simulink subsystem "rss_PwrTubPCBTempSensFaltDia"  (R2023a)
settings: Solver=VariableStepAuto  StartTime=0.0  StopTime=10.0  RelTol=1e-3
undefined symbols (not defined in the file): ENM_TYPE_FALT, Gu16_ctPCBTempFaltConfCnt_C, Gu16_ctPCBTempFaltRcvyCnt_C, Gu16_ctPwrTubTempFaltConfCnt_C, Gu16_ctPwrTubTempFaltRcvyCnt_C, Gu16_uADPCBTempFaltLoLim_C, Gu16_uADPwrTubTempFaltLoLim_C, Gu8_tNTCTempSensNoOpnCir_C, Gu8_tNTCTempSensOpnCir_C
libraries: lib_debounce x2, lib_configurable_parameter x2, lib_fault_definiteness x1
settings Model: Creator=xiaoqiang.yuan  LastModifiedBy=xiaoqiang.yuan

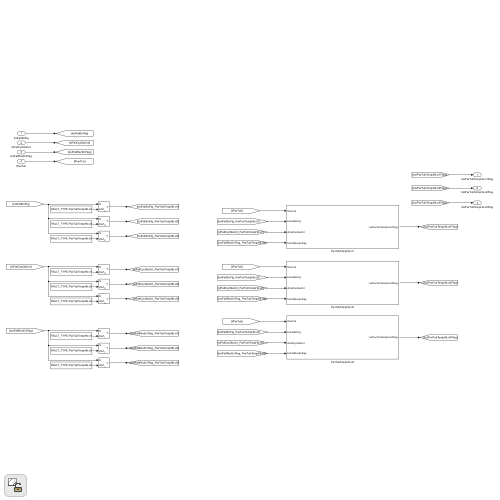
[thumbnail: Simulink's stored preview of the top-level diagram]
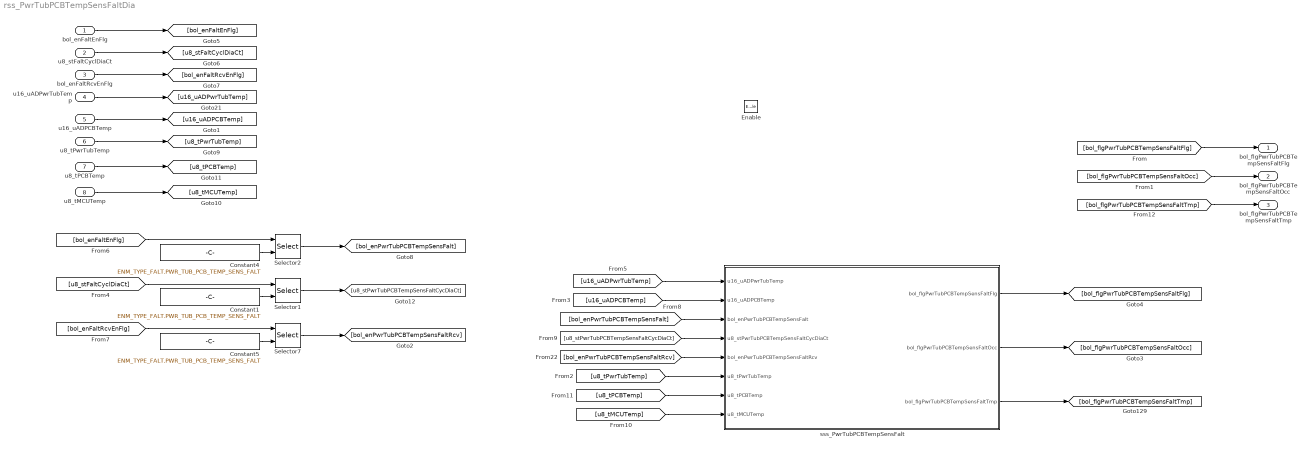
== system rss_PwrTubPCBTempSensFaltDia ==
  bol_enFaltEnFlg : Inport  OutDataTypeStr=boolean
  u8_stFaltCyclDiaCt : Inport  Port=2  OutDataTypeStr=uint8
  bol_enFaltRcvEnFlg : Inport  Port=3  OutDataTypeStr=boolean
  u16_uADPwrTubTemp : Inport  Port=4  OutDataTypeStr=uint16
  u16_uADPCBTemp : Inport  Port=5  OutDataTypeStr=uint16
  u8_tPwrTubTemp : Inport  Port=6  OutDataTypeStr=dt_Temp_u8p0bn40
  u8_tPCBTemp : Inport  Port=7  OutDataTypeStr=dt_Temp_u8p0bn40
  u8_tMCUTemp : Inport  Port=8  OutDataTypeStr=dt_Temp_u8p0bn40
  Enable : EnablePort
  Constant1 : Constant  Value=ENM_TYPE_FALT.PWR_TUB_PCB_TEMP_SENS_FALT
  Constant4 : Constant  Value=ENM_TYPE_FALT.PWR_TUB_PCB_TEMP_SENS_FALT
  Constant5 : Constant  Value=ENM_TYPE_FALT.PWR_TUB_PCB_TEMP_SENS_FALT
  Selector1 : Selector  IndexMode=Zero-based  InputPortWidth=Cdbl_numFaltDiaNum  IndexOptions=Index vector (port)  Indices=[1 3]  OutputSizes=1
  Selector2 : Selector  IndexMode=Zero-based  InputPortWidth=Cdbl_numFaltDiaNum  IndexOptions=Index vector (port)  Indices=[1 3]  OutputSizes=1
  Selector7 : Selector  IndexMode=Zero-based  InputPortWidth=Cdbl_numFaltDiaNum  IndexOptions=Index vector (port)  Indices=[1 3]  OutputSizes=1
  sss_PwrTubPCBTempSensFalt : Subsystem
  bol_flgPwrTubPCBTempSensFaltFlg : Outport  OutDataTypeStr=boolean
  bol_flgPwrTubPCBTempSensFaltOcc : Outport  Port=2  OutDataTypeStr=boolean
  bol_flgPwrTubPCBTempSensFaltTmp : Outport  Port=3  OutDataTypeStr=boolean
  wires:
  [bol_flgPwrTubPCBTempSensFaltFlg] -> bol_flgPwrTubPCBTempSensFaltFlg/1
  u16_uADPwrTubTemp/1 -> [u16_uADPwrTubTemp]
  Selector2/1 -> [bol_enPwrTubPCBTempSensFalt]
  [bol_enFaltEnFlg] -> Selector2/1
  [bol_enPwrTubPCBTempSensFalt] -> sss_PwrTubPCBTempSensFalt/3(bol_enPwrTubPCBTempSensFalt)
  Constant4/1 -> Selector2/2
  [u8_stPwrTubPCBTempSensFaltCycDiaCt] -> sss_PwrTubPCBTempSensFalt/4(u8_stPwrTubPCBTempSensFaltCycDiaCt)
  [u16_uADPwrTubTemp] -> sss_PwrTubPCBTempSensFalt/1(u16_uADPwrTubTemp)
  bol_enFaltEnFlg/1 -> [bol_enFaltEnFlg]
  bol_enFaltRcvEnFlg/1 -> [bol_enFaltRcvEnFlg]
  u8_stFaltCyclDiaCt/1 -> [u8_stFaltCyclDiaCt]
  [bol_enPwrTubPCBTempSensFaltRcv] -> sss_PwrTubPCBTempSensFalt/5(bol_enPwrTubPCBTempSensFaltRcv)
  Selector1/1 -> [u8_stPwrTubPCBTempSensFaltCycDiaCt]
  Constant1/1 -> Selector1/2
  [u8_stFaltCyclDiaCt] -> Selector1/1
  Selector7/1 -> [bol_enPwrTubPCBTempSensFaltRcv]
  Constant5/1 -> Selector7/2
  [bol_enFaltRcvEnFlg] -> Selector7/1
  sss_PwrTubPCBTempSensFalt/1(bol_flgPwrTubPCBTempSensFaltFlg) -> [bol_flgPwrTubPCBTempSensFaltFlg]
  u16_uADPCBTemp/1 -> [u16_uADPCBTemp]
  [u16_uADPCBTemp] -> sss_PwrTubPCBTempSensFalt/2(u16_uADPCBTemp)
  sss_PwrTubPCBTempSensFalt/2(bol_flgPwrTubPCBTempSensFaltOcc) -> [bol_flgPwrTubPCBTempSensFaltOcc]
  [bol_flgPwrTubPCBTempSensFaltOcc] -> bol_flgPwrTubPCBTempSensFaltOcc/1
  u8_tPCBTemp/1 -> [u8_tPCBTemp]
  u8_tMCUTemp/1 -> [u8_tMCUTemp]
  u8_tPwrTubTemp/1 -> [u8_tPwrTubTemp]
  [u8_tPwrTubTemp] -> sss_PwrTubPCBTempSensFalt/6(u8_tPwrTubTemp)
  [u8_tPCBTemp] -> sss_PwrTubPCBTempSensFalt/7(u8_tPCBTemp)
  [u8_tMCUTemp] -> sss_PwrTubPCBTempSensFalt/8(u8_tMCUTemp)
  [bol_flgPwrTubPCBTempSensFaltTmp] -> bol_flgPwrTubPCBTempSensFaltTmp/1
  sss_PwrTubPCBTempSensFalt/3(bol_flgPwrTubPCBTempSensFaltTmp) -> [bol_flgPwrTubPCBTempSensFaltTmp]

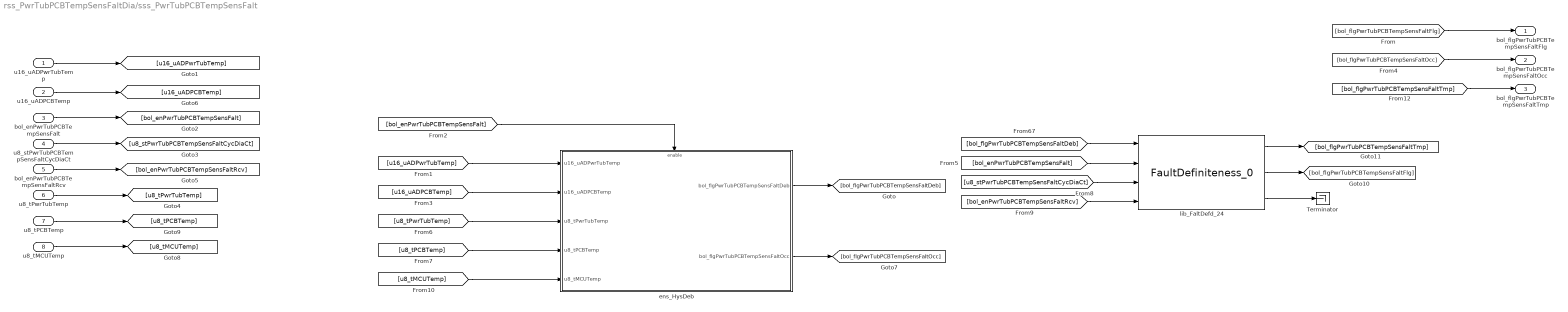
== system rss_PwrTubPCBTempSensFaltDia/sss_PwrTubPCBTempSensFalt ==
  u16_uADPwrTubTemp : Inport
  u16_uADPCBTemp : Inport  Port=2
  bol_enPwrTubPCBTempSensFalt : Inport  Port=3
  u8_stPwrTubPCBTempSensFaltCycDiaCt : Inport  Port=4
  bol_enPwrTubPCBTempSensFaltRcv : Inport  Port=5
  u8_tPwrTubTemp : Inport  Port=6
  u8_tPCBTemp : Inport  Port=7
  u8_tMCUTemp : Inport  Port=8
  Terminator : Terminator
  ens_HysDeb : Subsystem
  lib_FaltDefd_24 : lib_fault_definiteness/FaultDefiniteness_0  lb_FaltWaitRecvCnt=Gu16_ctPCBTempFaltConfCnt_C
  bol_flgPwrTubPCBTempSensFaltFlg : Outport
  bol_flgPwrTubPCBTempSensFaltOcc : Outport  Port=2
  bol_flgPwrTubPCBTempSensFaltTmp : Outport  Port=3  OutDataTypeStr=boolean
  wires:
  [bol_flgPwrTubPCBTempSensFaltTmp] -> bol_flgPwrTubPCBTempSensFaltTmp/1
  [u8_tMCUTemp] -> ens_HysDeb/5(u8_tMCUTemp)
  [u8_tPCBTemp] -> ens_HysDeb/4(u8_tPCBTemp)
  [u8_tPwrTubTemp] -> ens_HysDeb/3(u8_tPwrTubTemp)
  u8_tPCBTemp/1 -> [u8_tPCBTemp]
  u8_tPwrTubTemp/1 -> [u8_tPwrTubTemp]
  u8_tMCUTemp/1 -> [u8_tMCUTemp]
  [bol_flgPwrTubPCBTempSensFaltOcc] -> bol_flgPwrTubPCBTempSensFaltOcc/1
  ens_HysDeb/2(bol_flgPwrTubPCBTempSensFaltOcc) -> [bol_flgPwrTubPCBTempSensFaltOcc]
  [u16_uADPCBTemp] -> ens_HysDeb/2(u16_uADPCBTemp)
  u16_uADPCBTemp/1 -> [u16_uADPCBTemp]
  lib_FaltDefd_24/1 -> [bol_flgPwrTubPCBTempSensFaltTmp]
  lib_FaltDefd_24/2 -> [bol_flgPwrTubPCBTempSensFaltFlg]
  lib_FaltDefd_24/3 -> Terminator/1
  [bol_enPwrTubPCBTempSensFalt] -> ens_HysDeb/Enable
  [u16_uADPwrTubTemp] -> ens_HysDeb/1(u16_uADPwrTubTemp)
  ens_HysDeb/1(bol_flgPwrTubPCBTempSensFaltDeb) -> [bol_flgPwrTubPCBTempSensFaltDeb]
  bol_enPwrTubPCBTempSensFaltRcv/1 -> [bol_enPwrTubPCBTempSensFaltRcv]
  u8_stPwrTubPCBTempSensFaltCycDiaCt/1 -> [u8_stPwrTubPCBTempSensFaltCycDiaCt]
  bol_enPwrTubPCBTempSensFalt/1 -> [bol_enPwrTubPCBTempSensFalt]
  [bol_flgPwrTubPCBTempSensFaltFlg] -> bol_flgPwrTubPCBTempSensFaltFlg/1
  u16_uADPwrTubTemp/1 -> [u16_uADPwrTubTemp]
  [bol_enPwrTubPCBTempSensFaltRcv] -> lib_FaltDefd_24/4
  [u8_stPwrTubPCBTempSensFaltCycDiaCt] -> lib_FaltDefd_24/3
  [bol_enPwrTubPCBTempSensFalt] -> lib_FaltDefd_24/2
  [bol_flgPwrTubPCBTempSensFaltDeb] -> lib_FaltDefd_24/1

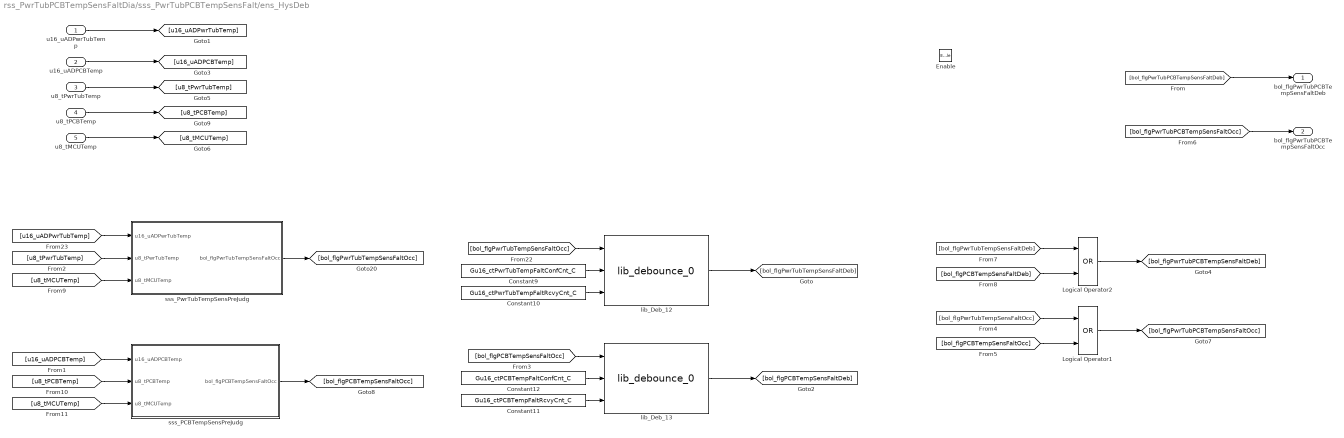
== system rss_PwrTubPCBTempSensFaltDia/sss_PwrTubPCBTempSensFalt/ens_HysDeb ==
  u16_uADPwrTubTemp : Inport
  u16_uADPCBTemp : Inport  Port=2
  u8_tPwrTubTemp : Inport  Port=3
  u8_tPCBTemp : Inport  Port=4
  u8_tMCUTemp : Inport  Port=5
  Enable : EnablePort
  Constant10 : Constant  Value=Gu16_ctPwrTubTempFaltRcvyCnt_C
  Constant11 : Constant  Value=Gu16_ctPCBTempFaltRcvyCnt_C
  Constant12 : Constant  Value=Gu16_ctPCBTempFaltConfCnt_C
  Constant9 : Constant  Value=Gu16_ctPwrTubTempFaltConfCnt_C
  Logical Operator1 : Logic  Operator=OR  AllPortsSameDT=off  OutDataTypeStr=boolean
  Logical Operator2 : Logic  Operator=OR  AllPortsSameDT=off  OutDataTypeStr=boolean
  lib_Deb_12 : lib_debounce/lib_debounce_0
  lib_Deb_13 : lib_debounce/lib_debounce_0
  sss_PCBTempSensPreJudg : Subsystem
  sss_PwrTubTempSensPreJudg : Subsystem
  bol_flgPwrTubPCBTempSensFaltDeb : Outport
  bol_flgPwrTubPCBTempSensFaltOcc : Outport  Port=2
  wires:
  [u8_tMCUTemp] -> sss_PCBTempSensPreJudg/3(u8_tMCUTemp)
  [u8_tPCBTemp] -> sss_PCBTempSensPreJudg/2(u8_tPCBTemp)
  [u8_tMCUTemp] -> sss_PwrTubTempSensPreJudg/3(u8_tMCUTemp)
  [u8_tPwrTubTemp] -> sss_PwrTubTempSensPreJudg/2(u8_tPwrTubTemp)
  u8_tPCBTemp/1 -> [u8_tPCBTemp]
  u8_tMCUTemp/1 -> [u8_tMCUTemp]
  u8_tPwrTubTemp/1 -> [u8_tPwrTubTemp]
  Logical Operator2/1 -> [bol_flgPwrTubPCBTempSensFaltDeb]
  [bol_flgPwrTubTempSensFaltDeb] -> Logical Operator2/1
  [bol_flgPCBTempSensFaltDeb] -> Logical Operator2/2
  sss_PCBTempSensPreJudg/1(bol_flgPCBTempSensFaltOcc) -> [bol_flgPCBTempSensFaltOcc]
  [bol_flgPCBTempSensFaltOcc] -> lib_Deb_13/1
  lib_Deb_13/1 -> [bol_flgPCBTempSensFaltDeb]
  Constant11/1 -> lib_Deb_13/3
  Constant12/1 -> lib_Deb_13/2
  [u16_uADPCBTemp] -> sss_PCBTempSensPreJudg/1(u16_uADPCBTemp)
  lib_Deb_12/1 -> [bol_flgPwrTubTempSensFaltDeb]
  [bol_flgPwrTubTempSensFaltOcc] -> lib_Deb_12/1
  Constant9/1 -> lib_Deb_12/2
  sss_PwrTubTempSensPreJudg/1(bol_flgPwrTubTempSensFaltOcc) -> [bol_flgPwrTubTempSensFaltOcc]
  Constant10/1 -> lib_Deb_12/3
  [u16_uADPwrTubTemp] -> sss_PwrTubTempSensPreJudg/1(u16_uADPwrTubTemp)
  [bol_flgPwrTubPCBTempSensFaltOcc] -> bol_flgPwrTubPCBTempSensFaltOcc/1
  Logical Operator1/1 -> [bol_flgPwrTubPCBTempSensFaltOcc]
  [bol_flgPCBTempSensFaltOcc] -> Logical Operator1/2
  [bol_flgPwrTubTempSensFaltOcc] -> Logical Operator1/1
  u16_uADPCBTemp/1 -> [u16_uADPCBTemp]
  u16_uADPwrTubTemp/1 -> [u16_uADPwrTubTemp]
  [bol_flgPwrTubPCBTempSensFaltDeb] -> bol_flgPwrTubPCBTempSensFaltDeb/1

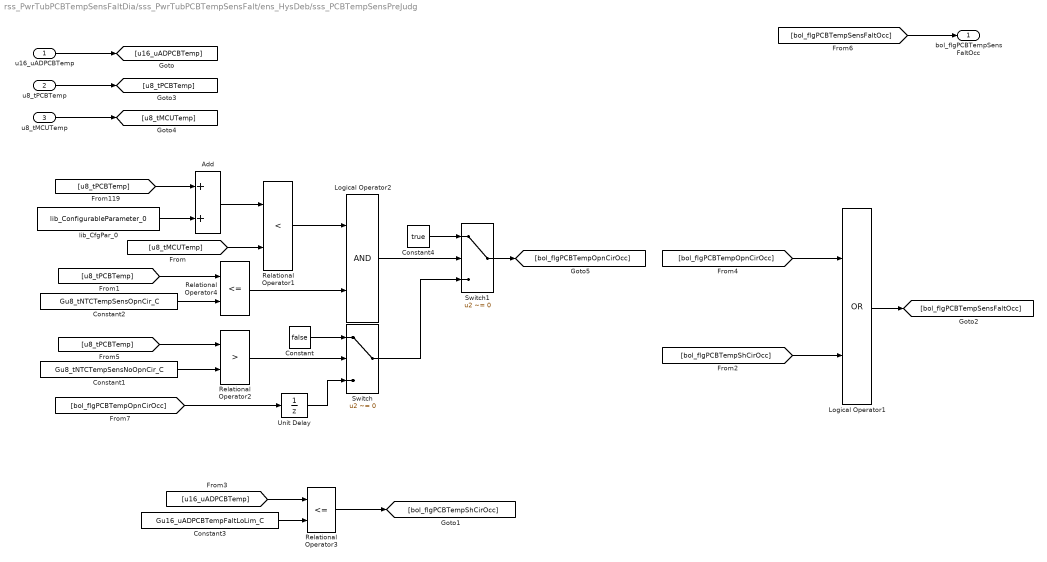
== system rss_PwrTubPCBTempSensFaltDia/sss_PwrTubPCBTempSensFalt/ens_HysDeb/sss_PCBTempSensPreJudg ==
  u16_uADPCBTemp : Inport
  u8_tPCBTemp : Inport  Port=2
  u8_tMCUTemp : Inport  Port=3
  Add : Sum  OutDataTypeStr=Inherit: Same as first input
  Constant : Constant  Value=false  OutDataTypeStr=boolean
  Constant1 : Constant  Value=Gu8_tNTCTempSensNoOpnCir_C
  Constant2 : Constant  Value=Gu8_tNTCTempSensOpnCir_C
  Constant3 : Constant  Value=Gu16_uADPCBTempFaltLoLim_C
  Constant4 : Constant  Value=true  OutDataTypeStr=boolean
  Logical Operator1 : Logic  Operator=OR  AllPortsSameDT=off  OutDataTypeStr=boolean
  Logical Operator2 : Logic  AllPortsSameDT=off  OutDataTypeStr=boolean
  Relational Operator1 : RelationalOperator  Operator=<  OutDataTypeStr=boolean  RndMeth=Simplest  InputSameDT=off
  Relational Operator2 : RelationalOperator  Operator=>  OutDataTypeStr=boolean  RndMeth=Simplest  InputSameDT=off
  Relational Operator3 : RelationalOperator  Operator=<=  OutDataTypeStr=boolean  RndMeth=Simplest  InputSameDT=off
  Relational Operator4 : RelationalOperator  Operator=<=  OutDataTypeStr=boolean  RndMeth=Simplest  InputSameDT=off
  Switch : Switch  Criteria=u2 ~= 0  SaturateOnIntegerOverflow=off  InputSameDT=off  OutDataTypeStr=Inherit: Same as first input
  Switch1 : Switch  Criteria=u2 ~= 0  SaturateOnIntegerOverflow=off  InputSameDT=off  OutDataTypeStr=Inherit: Same as first input
  Unit Delay : UnitDelay  InitialCondition=boolean(0)  SampleTime=-1  HasFrameUpgradeWarning=on
  lib_CfgPar_0 : lib_configurable_parameter/lib_ConfigurableParameter_0  lb_parCnfgPar=Gu8_tMaxNTCMCUTempDvt_C  lb_parDataType=Inherit: Inherit from 'Constant value'  lb_parUpLim=Cdbl_tNTCMCUTempDvtMaxVal  lb_parLowLim=0
  bol_flgPCBTempSensFaltOcc : Outport
  wires:
  Unit Delay/1 -> Switch/3
  [bol_flgPCBTempOpnCirOcc] -> Unit Delay/1
  Switch1/1 -> [bol_flgPCBTempOpnCirOcc]
  Switch/1 -> Switch1/3
  Constant4/1 -> Switch1/1
  Logical Operator2/1 -> Switch1/2
  Relational Operator2/1 -> Switch/2
  Constant/1 -> Switch/1
  [u8_tPCBTemp] -> Relational Operator2/1
  Constant1/1 -> Relational Operator2/2
  [bol_flgPCBTempOpnCirOcc] -> Logical Operator1/1
  [bol_flgPCBTempShCirOcc] -> Logical Operator1/2
  Relational Operator3/1 -> [bol_flgPCBTempShCirOcc]
  u8_tMCUTemp/1 -> [u8_tMCUTemp]
  u8_tPCBTemp/1 -> [u8_tPCBTemp]
  [u8_tMCUTemp] -> Relational Operator1/2
  [u8_tPCBTemp] -> Relational Operator4/1
  lib_CfgPar_0/1 -> Add/2
  Constant2/1 -> Relational Operator4/2
  Relational Operator1/1 -> Logical Operator2/1
  Add/1 -> Relational Operator1/1
  [u8_tPCBTemp] -> Add/1
  Constant3/1 -> Relational Operator3/2
  Logical Operator1/1 -> [bol_flgPCBTempSensFaltOcc]
  [u16_uADPCBTemp] -> Relational Operator3/1
  Relational Operator4/1 -> Logical Operator2/2
  u16_uADPCBTemp/1 -> [u16_uADPCBTemp]
  [bol_flgPCBTempSensFaltOcc] -> bol_flgPCBTempSensFaltOcc/1

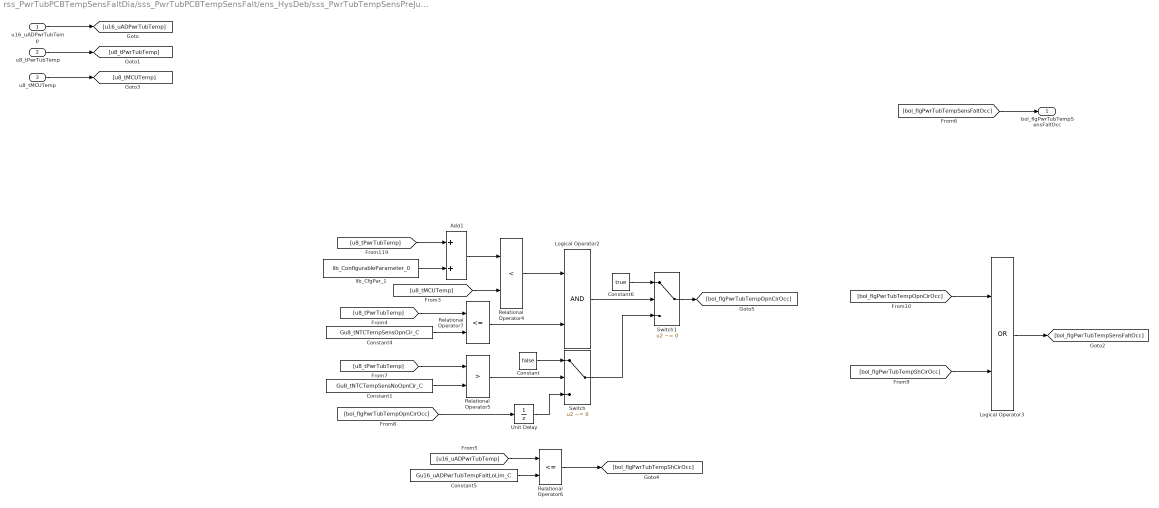
== system rss_PwrTubPCBTempSensFaltDia/sss_PwrTubPCBTempSensFalt/ens_HysDeb/sss_PwrTubTempSensPreJudg ==
  u16_uADPwrTubTemp : Inport
  u8_tPwrTubTemp : Inport  Port=2
  u8_tMCUTemp : Inport  Port=3
  Add1 : Sum  OutDataTypeStr=Inherit: Same as first input
  Constant : Constant  Value=false  OutDataTypeStr=boolean
  Constant1 : Constant  Value=Gu8_tNTCTempSensNoOpnCir_C
  Constant4 : Constant  Value=Gu8_tNTCTempSensOpnCir_C
  Constant5 : Constant  Value=Gu16_uADPwrTubTempFaltLoLim_C
  Constant6 : Constant  Value=true  OutDataTypeStr=boolean
  Logical Operator2 : Logic  AllPortsSameDT=off  OutDataTypeStr=boolean
  Logical Operator3 : Logic  Operator=OR  AllPortsSameDT=off  OutDataTypeStr=boolean
  Relational Operator4 : RelationalOperator  Operator=<  OutDataTypeStr=boolean  RndMeth=Simplest  InputSameDT=off
  Relational Operator5 : RelationalOperator  Operator=>  OutDataTypeStr=boolean  RndMeth=Simplest  InputSameDT=off
  Relational Operator6 : RelationalOperator  Operator=<=  OutDataTypeStr=boolean  RndMeth=Simplest  InputSameDT=off
  Relational Operator7 : RelationalOperator  Operator=<=  OutDataTypeStr=boolean  RndMeth=Simplest  InputSameDT=off
  Switch : Switch  Criteria=u2 ~= 0  SaturateOnIntegerOverflow=off  InputSameDT=off  OutDataTypeStr=Inherit: Same as first input
  Switch1 : Switch  Criteria=u2 ~= 0  SaturateOnIntegerOverflow=off  InputSameDT=off  OutDataTypeStr=Inherit: Same as first input
  Unit Delay : UnitDelay  InitialCondition=boolean(0)  SampleTime=-1  HasFrameUpgradeWarning=on
  lib_CfgPar_1 : lib_configurable_parameter/lib_ConfigurableParameter_0  lb_parCnfgPar=Gu8_tMaxNTCMCUTempDvt_C  lb_parDataType=Inherit: Inherit from 'Constant value'  lb_parUpLim=Cdbl_tNTCMCUTempDvtMaxVal  lb_parLowLim=0
  bol_flgPwrTubTempSensFaltOcc : Outport
  wires:
  Logical Operator3/1 -> [bol_flgPwrTubTempSensFaltOcc]
  [bol_flgPwrTubTempSensFaltOcc] -> bol_flgPwrTubTempSensFaltOcc/1
  [bol_flgPwrTubTempShCirOcc] -> Logical Operator3/2
  [bol_flgPwrTubTempOpnCirOcc] -> Logical Operator3/1
  [u8_tPwrTubTemp] -> Relational Operator7/1
  [u8_tMCUTemp] -> Relational Operator4/2
  [u16_uADPwrTubTemp] -> Relational Operator6/1
  [u8_tPwrTubTemp] -> Add1/1
  lib_CfgPar_1/1 -> Add1/2
  Relational Operator4/1 -> Logical Operator2/1
  Add1/1 -> Relational Operator4/1
  Constant1/1 -> Relational Operator5/2
  Constant4/1 -> Relational Operator7/2
  Relational Operator7/1 -> Logical Operator2/2
  Constant5/1 -> Relational Operator6/2
  Constant6/1 -> Switch1/1
  [u8_tPwrTubTemp] -> Relational Operator5/1
  Logical Operator2/1 -> Switch1/2
  Switch/1 -> Switch1/3
  [bol_flgPwrTubTempOpnCirOcc] -> Unit Delay/1
  Switch1/1 -> [bol_flgPwrTubTempOpnCirOcc]
  Unit Delay/1 -> Switch/3
  Relational Operator5/1 -> Switch/2
  Relational Operator6/1 -> [bol_flgPwrTubTempShCirOcc]
  Constant/1 -> Switch/1
  u8_tMCUTemp/1 -> [u8_tMCUTemp]
  u8_tPwrTubTemp/1 -> [u8_tPwrTubTemp]
  u16_uADPwrTubTemp/1 -> [u16_uADPwrTubTemp]
